simulink model "slidemodel"  (Simulink 8.5)
settings: Solver=ode45  StartTime=0.0  StopTime=10  FixedStep=0.01  RelTol=1e-3
settings Model: Creator=hp  LastModifiedBy=18813  ExtModeTrigMode=oneshot  ExtModeArmWhenConnect=off
settings DataIOCC: LimitDataPoints=off  SignalLoggingName=sigsOut
settings OptimizationCC: BooleanDataType=off  InitFltsAndDblsToZero=on
settings DebuggingCC: SaveWithParameterizedLinksMsg=none  SignalResolutionControl=TryResolveAllWithWarning  MultiTaskDSMMsg=warning  MultiTaskCondExecSysMsg=none  FcnCallInpInsideContextMsg=UseLocalSettings
settings HardwareCC: TargetUnknown=on
settings GRTTargetCC: TargetFcnLib=ansi_tfl_tmw.mat

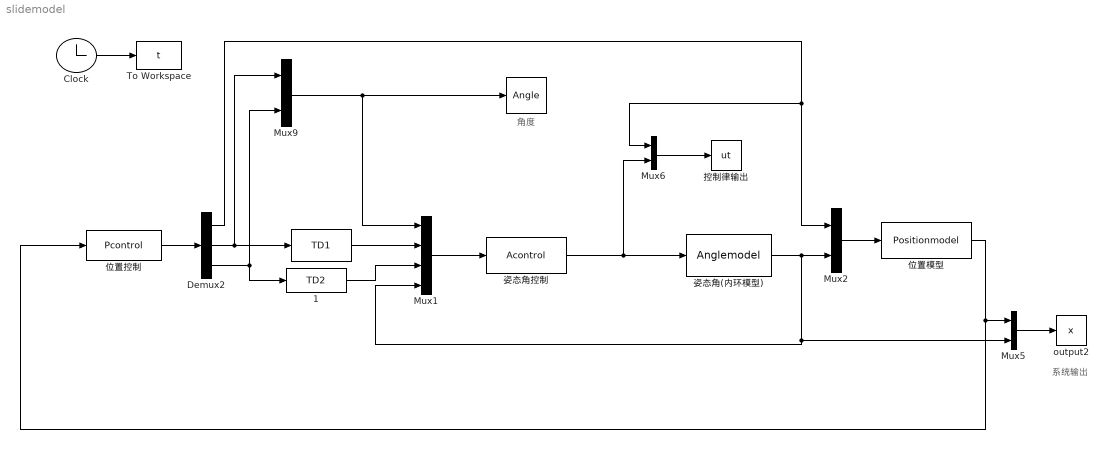
== system slidemodel ==
  note: 系统输出
  note: 角度
  " " : S-Function  FunctionName=TD1
  "   " : ToWorkspace  VariableName=Angle  SampleTime=-1
  " 1" : S-Function  FunctionName=TD2
  Clock : Clock
  Demux2 : Demux  Outputs=3
  Mux1 : Mux
  Mux{2,5..6,9} (4 alike) : Mux  Inputs=2
  To Workspace : ToWorkspace  VariableName=t  SampleTime=-1
  output2 : ToWorkspace  VariableName=x  SampleTime=-1
  位置控制 : S-Function  FunctionName=Pcontrol
  位置模型 : S-Function  FunctionName=Positionmodel
  姿态角(内环模型) : S-Function  FunctionName=Anglemodel
  姿态角控制 : S-Function  FunctionName=Acontrol
  控制律输出 : ToWorkspace  VariableName=ut  SampleTime=-1
  wires:
  Clock/1 -> To Workspace/1
  位置控制/1 -> Demux2/1
  Demux2/3 -> Mux9/2, " 1"/1
  Demux2/2 -> Mux9/1, " "/1
  Mux1/1 -> 姿态角控制/1
  Mux9/1 -> Mux1/1, "   "/1
  Mux6/1 -> 控制律输出/1
  姿态角控制/1 -> Mux6/2, 姿态角(内环模型)/1
  Mux2/1 -> 位置模型/1
  姿态角(内环模型)/1 -> Mux5/2, Mux1/4, Mux2/2
  Demux2/1 -> Mux2/1, Mux6/1
  " "/1 -> Mux1/2
  " 1"/1 -> Mux1/3
  Mux5/1 -> output2/1
  位置模型/1 -> Mux5/1, 位置控制/1
